simulink model "ThdRwLtStCaller"  (R2018b)
settings: Solver=FixedStepDiscrete  StartTime=0.0  StopTime=10.0  RelTol=1e-3
undefined symbols (not defined in the file): ThdRwLtStBkReclnCtrl_1_Cal, ThdRwLtStBkReclnHolderChk_1_Cal, ThdRwLtStBkReclnIsPosChk_1_Cal, ThdRwLtStBkReclnTrgtPosSelc_1_Cal, ThdRwLtStCshnFldCtrl_1_Cal, ThdRwLtStCshnFldHolderChk_1_Cal, ThdRwLtStCshnFldIsPosChk_1_Cal, ThdRwLtStCshnFldTrgtPosSelc_1_Cal, ThdRwLtStFwdBkwdCtrl_1_Cal, ThdRwLtStFwdBkwdHolderChk_1_Cal, ThdRwLtStFwdBkwdIsPosChk_1_Cal, ThdRwLtStFwdBkwdSpdCtrl_1_Cal, ThdRwLtStFwdBkwdTrgtPosSelc_1_Cal, ThdRwLtStRclCmdSrvCal_1_Cal
settings Model: Creator=sn2xws  LastModifiedBy=sn2xws
settings DataIOCC: SaveFormat=StructureWithTime
settings OptimizationCC: DefaultParameterBehavior=Inlined  EnhancedBackFolding=on  PassReuseOutputArgsAs=Individual arguments  ZeroExternalMemoryAtStartup=off  ZeroInternalMemoryAtStartup=off  OptimizeBlockOrder=speed  DifferentSizesBufferReuse=on  OptimizationCustomize=off
settings DebuggingCC: ParameterTunabilityLossMsg=error
settings SFSimCC: MATLABDynamicMemAlloc=off
settings RTWCC: SystemTargetFile=autosar.tlc  GenCodeOnly=on  TemplateMakefile=ert_default_tmf  Description=AUTOSAR  GenerateReport=on  IncludeHyperlinkInReport=on  LaunchReport=on  GenerateTraceInfo=on  GenerateTraceReport=on  GenerateTraceReportSl=on  GenerateTraceReportSf=on  GenerateTraceReportEml=on  GenerateCodeMetricsReport=on
settings CodeAppCC: ForceParamTrailComments=on  IgnoreCustomStorageClasses=off  OperatorAnnotations=on  SimulinkDataObjDesc=on  SFDataObjDesc=on  InsertBlockDesc=on
settings STFCustomTargetCC: TargetLangStandard=C99 (ISO)  MultiwordLength=256  ParMdlRefBuildCompliant=on  CompOptLevelCompliant=on  IncludeMdlTerminateFcn=off  CombineOutputUpdateFcns=on  SuppressErrorStatus=on  ERTCustomFileBanners=on  SupportNonFinite=off  SupportComplex=off  SupportContinuousTime=off  SupportNonInlinedSFcns=off  RemoveResetFunc=on  MATLABClassNameForMDSCustomization=Simulink.SoftwareTarget.ERTCustomization  AutosarCompliant=on  UseToolchainInfoCompliant=on  LookupTableObjectStructAxisOrder=2,1,3,4,...  LUTObjectStructOrderEvenSpacing=Size,Table,Breakpoints  SystemTargetFile=autosar.tlc
settings ERTTargetCC: TargetLangStandard=C99 (ISO)  ConcurrentExecutionCompliant=off  IncludeMdlTerminateFcn=off  SuppressErrorStatus=on  SupportNonFinite=off  SupportComplex=off  ModelStepFunctionPrototypeControlCompliant=off  CPPClassGenCompliant=off  AutosarCompliant=on  LookupTableObjectStructAxisOrder=2,1,3,4,...  LUTObjectStructOrderEvenSpacing=Size,Table,Breakpoints  InlinedParameterPlacement=NonHierarchical  ERTCustomFileTemplate=example_file_process.tlc  ERTFilePackagingFormat=Compact

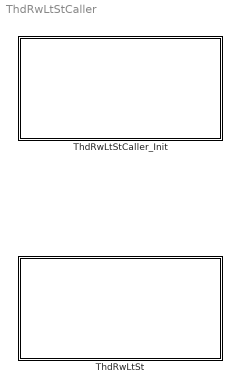
== system ThdRwLtStCaller ==
  ThdRwLtSt : Subsystem
  ThdRwLtStCaller_Init : Subsystem

== system ThdRwLtStCaller/ThdRwLtSt ==
  ThdRwLtSt_Cal_sys : Subsystem

== system ThdRwLtStCaller/ThdRwLtStCaller_Init ==
  Event Listener : EventListener  EventName=reset

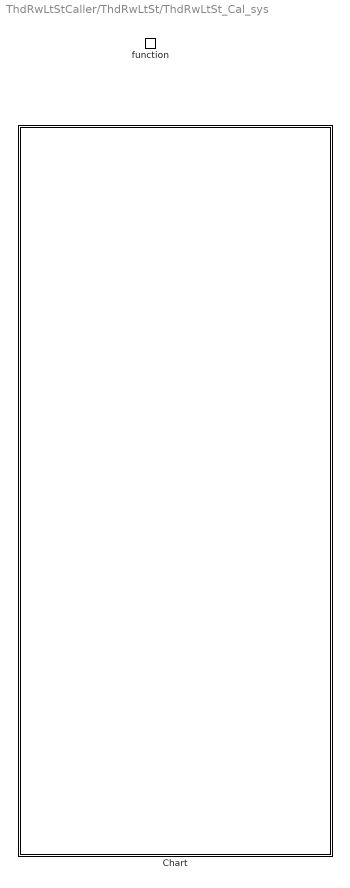
== system ThdRwLtStCaller/ThdRwLtSt/ThdRwLtSt_Cal_sys ==
  function : TriggerPort  TriggerType=function-call  IsSimulinkFunction=on  FunctionName=ThdRwLtSt_Cal  VariantControl=(inherit)
  Chart : Stateflow chart  TreatAsAtomicUnit=on

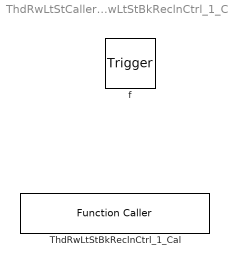
== system ThdRwLtStCaller/ThdRwLtSt/ThdRwLtSt_Cal_sys/Chart/ThdRwLtStBkReclnCtrl_1_Cal ==
  f : TriggerPort  TriggerType=function-call  VariantControl=(inherit)
      settings: CopyFcn=Stateflow.SLINSF.SimulinkMan.removeBlockPreDeleteFcn  PreDeleteFcn=Stateflow.SLINSF.SimulinkMan.unsafePredeleteFcn
  ThdRwLtStBkReclnCtrl_1_Cal : FunctionCaller  FunctionPrototype=ThdRwLtStBkReclnCtrl_1_Cal()

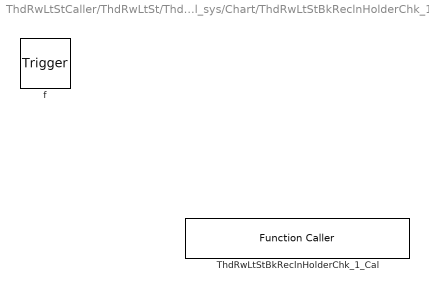
== system ThdRwLtStCaller/ThdRwLtSt/ThdRwLtSt_Cal_sys/Chart/ThdRwLtStBkReclnHolderChk_1_Cal ==
  f : TriggerPort  TriggerType=function-call  VariantControl=(inherit)
      settings: CopyFcn=Stateflow.SLINSF.SimulinkMan.removeBlockPreDeleteFcn  PreDeleteFcn=Stateflow.SLINSF.SimulinkMan.unsafePredeleteFcn
  ThdRwLtStBkReclnHolderChk_1_Cal : FunctionCaller  FunctionPrototype=ThdRwLtStBkReclnHolderChk_1_Cal()

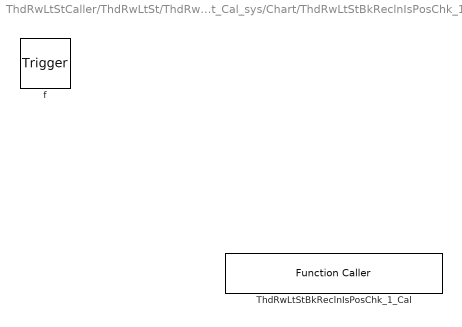
== system ThdRwLtStCaller/ThdRwLtSt/ThdRwLtSt_Cal_sys/Chart/ThdRwLtStBkReclnIsPosChk_1_Cal ==
  f : TriggerPort  TriggerType=function-call  VariantControl=(inherit)
      settings: CopyFcn=Stateflow.SLINSF.SimulinkMan.removeBlockPreDeleteFcn  PreDeleteFcn=Stateflow.SLINSF.SimulinkMan.unsafePredeleteFcn
  ThdRwLtStBkReclnIsPosChk_1_Cal : FunctionCaller  FunctionPrototype=ThdRwLtStBkReclnIsPosChk_1_Cal()

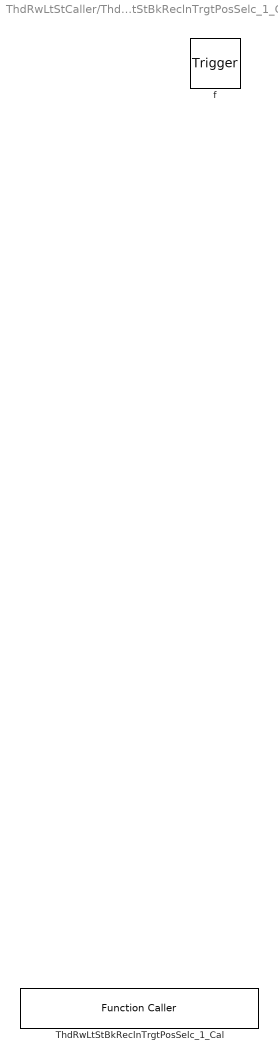
== system ThdRwLtStCaller/ThdRwLtSt/ThdRwLtSt_Cal_sys/Chart/ThdRwLtStBkReclnTrgtPosSelc_1_Cal ==
  f : TriggerPort  TriggerType=function-call  VariantControl=(inherit)
      settings: CopyFcn=Stateflow.SLINSF.SimulinkMan.removeBlockPreDeleteFcn  PreDeleteFcn=Stateflow.SLINSF.SimulinkMan.unsafePredeleteFcn
  ThdRwLtStBkReclnTrgtPosSelc_1_Cal : FunctionCaller  FunctionPrototype=ThdRwLtStBkReclnTrgtPosSelc_1_Cal()

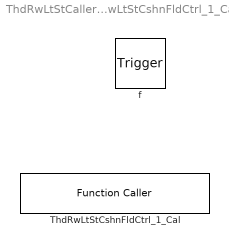
== system ThdRwLtStCaller/ThdRwLtSt/ThdRwLtSt_Cal_sys/Chart/ThdRwLtStCshnFldCtrl_1_Cal ==
  f : TriggerPort  TriggerType=function-call  VariantControl=(inherit)
      settings: CopyFcn=Stateflow.SLINSF.SimulinkMan.removeBlockPreDeleteFcn  PreDeleteFcn=Stateflow.SLINSF.SimulinkMan.unsafePredeleteFcn
  ThdRwLtStCshnFldCtrl_1_Cal : FunctionCaller  FunctionPrototype=ThdRwLtStCshnFldCtrl_1_Cal()

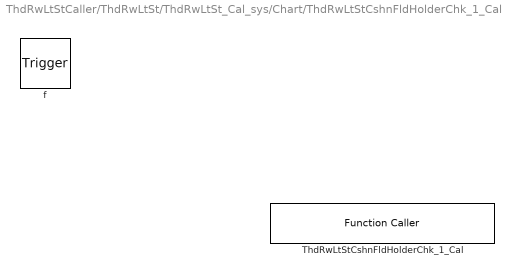
== system ThdRwLtStCaller/ThdRwLtSt/ThdRwLtSt_Cal_sys/Chart/ThdRwLtStCshnFldHolderChk_1_Cal ==
  f : TriggerPort  TriggerType=function-call  VariantControl=(inherit)
      settings: CopyFcn=Stateflow.SLINSF.SimulinkMan.removeBlockPreDeleteFcn  PreDeleteFcn=Stateflow.SLINSF.SimulinkMan.unsafePredeleteFcn
  ThdRwLtStCshnFldHolderChk_1_Cal : FunctionCaller  FunctionPrototype=ThdRwLtStCshnFldHolderChk_1_Cal()

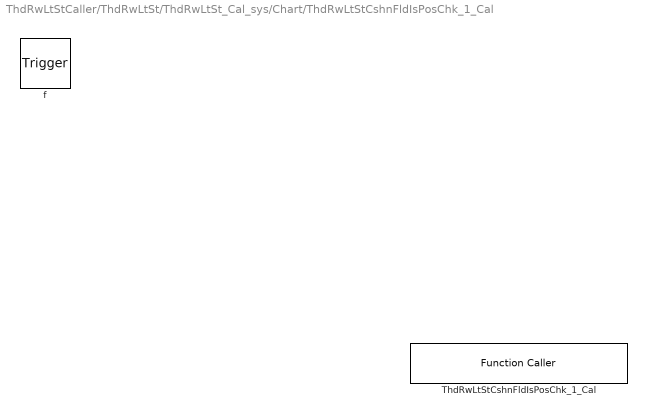
== system ThdRwLtStCaller/ThdRwLtSt/ThdRwLtSt_Cal_sys/Chart/ThdRwLtStCshnFldIsPosChk_1_Cal ==
  f : TriggerPort  TriggerType=function-call  VariantControl=(inherit)
      settings: CopyFcn=Stateflow.SLINSF.SimulinkMan.removeBlockPreDeleteFcn  PreDeleteFcn=Stateflow.SLINSF.SimulinkMan.unsafePredeleteFcn
  ThdRwLtStCshnFldIsPosChk_1_Cal : FunctionCaller  FunctionPrototype=ThdRwLtStCshnFldIsPosChk_1_Cal()

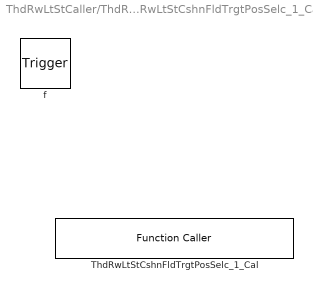
== system ThdRwLtStCaller/ThdRwLtSt/ThdRwLtSt_Cal_sys/Chart/ThdRwLtStCshnFldTrgtPosSelc_1_Cal ==
  f : TriggerPort  TriggerType=function-call  VariantControl=(inherit)
      settings: CopyFcn=Stateflow.SLINSF.SimulinkMan.removeBlockPreDeleteFcn  PreDeleteFcn=Stateflow.SLINSF.SimulinkMan.unsafePredeleteFcn
  ThdRwLtStCshnFldTrgtPosSelc_1_Cal : FunctionCaller  FunctionPrototype=ThdRwLtStCshnFldTrgtPosSelc_1_Cal()

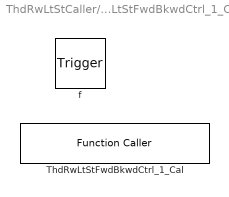
== system ThdRwLtStCaller/ThdRwLtSt/ThdRwLtSt_Cal_sys/Chart/ThdRwLtStFwdBkwdCtrl_1_Cal ==
  f : TriggerPort  TriggerType=function-call  VariantControl=(inherit)
      settings: CopyFcn=Stateflow.SLINSF.SimulinkMan.removeBlockPreDeleteFcn  PreDeleteFcn=Stateflow.SLINSF.SimulinkMan.unsafePredeleteFcn
  ThdRwLtStFwdBkwdCtrl_1_Cal : FunctionCaller  FunctionPrototype=ThdRwLtStFwdBkwdCtrl_1_Cal()

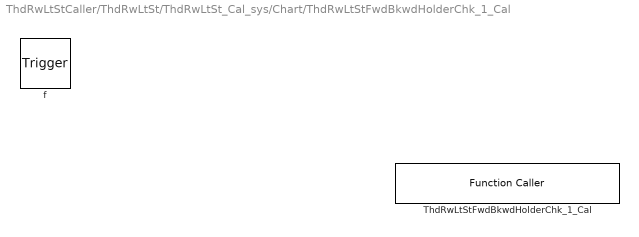
== system ThdRwLtStCaller/ThdRwLtSt/ThdRwLtSt_Cal_sys/Chart/ThdRwLtStFwdBkwdHolderChk_1_Cal ==
  f : TriggerPort  TriggerType=function-call  VariantControl=(inherit)
      settings: CopyFcn=Stateflow.SLINSF.SimulinkMan.removeBlockPreDeleteFcn  PreDeleteFcn=Stateflow.SLINSF.SimulinkMan.unsafePredeleteFcn
  ThdRwLtStFwdBkwdHolderChk_1_Cal : FunctionCaller  FunctionPrototype=ThdRwLtStFwdBkwdHolderChk_1_Cal()

== system ThdRwLtStCaller/ThdRwLtSt/ThdRwLtSt_Cal_sys/Chart/ThdRwLtStFwdBkwdIsPosChk_1_Cal ==
  f : TriggerPort  TriggerType=function-call  VariantControl=(inherit)
      settings: CopyFcn=Stateflow.SLINSF.SimulinkMan.removeBlockPreDeleteFcn  PreDeleteFcn=Stateflow.SLINSF.SimulinkMan.unsafePredeleteFcn
  ThdRwLtStFwdBkwdIsPosChk_1_Cal : FunctionCaller  FunctionPrototype=ThdRwLtStFwdBkwdIsPosChk_1_Cal()

== system ThdRwLtStCaller/ThdRwLtSt/ThdRwLtSt_Cal_sys/Chart/ThdRwLtStFwdBkwdSpdCtrl_1_Cal ==
  f : TriggerPort  TriggerType=function-call  VariantControl=(inherit)
      settings: CopyFcn=Stateflow.SLINSF.SimulinkMan.removeBlockPreDeleteFcn  PreDeleteFcn=Stateflow.SLINSF.SimulinkMan.unsafePredeleteFcn
  ThdRwLtStFwdBkwdSpdCtrl_1_Cal : FunctionCaller  FunctionPrototype=ThdRwLtStFwdBkwdSpdCtrl_1_Cal()

== system ThdRwLtStCaller/ThdRwLtSt/ThdRwLtSt_Cal_sys/Chart/ThdRwLtStFwdBkwdTrgtPosSelc_1_Cal ==
  f : TriggerPort  TriggerType=function-call  VariantControl=(inherit)
      settings: CopyFcn=Stateflow.SLINSF.SimulinkMan.removeBlockPreDeleteFcn  PreDeleteFcn=Stateflow.SLINSF.SimulinkMan.unsafePredeleteFcn
  ThdRwLtStFwdBkwdTrgtPosSelc_1_Cal : FunctionCaller  FunctionPrototype=ThdRwLtStFwdBkwdTrgtPosSelc_1_Cal()

== system ThdRwLtStCaller/ThdRwLtSt/ThdRwLtSt_Cal_sys/Chart/ThdRwLtStRclCmdSrvCal_1_Cal ==
  f : TriggerPort  TriggerType=function-call  VariantControl=(inherit)
      settings: CopyFcn=Stateflow.SLINSF.SimulinkMan.removeBlockPreDeleteFcn  PreDeleteFcn=Stateflow.SLINSF.SimulinkMan.unsafePredeleteFcn
  ThdRwLtStRclCmdSrvCal_1_Cal : FunctionCaller  FunctionPrototype=ThdRwLtStRclCmdSrvCal_1_Cal()

== stateflow chart ThdRwLtStCaller/ThdRwLtSt/ThdRwLtSt_Cal_sys/Chart ==
  state ThdRwLtStBkReclnTrgtPosSelc_1_Cal [function]
  state ThdRwLtStCshnFldTrgtPosSelc_1_Cal [function]
  state ThdRwLtStFwdBkwdTrgtPosSelc_1_Cal [function]
  state ThdRwLtStBkReclnIsPosChk_1_Cal [function]
  state ThdRwLtStCshnFldIsPosChk_1_Cal [function]
  state ThdRwLtStFwdBkwdIsPosChk_1_Cal [function]
  state ThdRwLtStBkReclnHolderChk_1_Cal [function]
  state ThdRwLtStCshnFldHolderChk_1_Cal [function]
  state ThdRwLtStFwdBkwdHolderChk_1_Cal [function]
  state ThdRwLtStBkReclnCtrl_1_Cal [function]
  state ThdRwLtStCshnFldCtrl_1_Cal [function]
  state ThdRwLtStFwdBkwdCtrl_1_Cal [function]
  state ThdRwLtStFwdBkwdSpdCtrl_1_Cal [function]
  state ThdRwLtStRclCmdSrvCal_1_Cal [function]
  (default) -> (junction 15)
  (junction 15) -> (junction 17) : {
      | ThdRwLtStBkReclnTrgtPosSelc_1_Cal();
      | ThdRwLtStCshnFldTrgtPosSelc_1_Cal();
      | ThdRwLtStFwdBkwdTrgtPosSelc_1_Cal();
      | ThdRwLtStBkReclnIsPosChk_1_Cal();
      | ThdRwLtStCshnFldIsPosChk_1_Cal();
      | ThdRwLtStFwdBkwdIsPosChk_1_Cal();
      | ThdRwLtStBkReclnHolderChk_1_Cal();
      | ThdRwLtStCshnFldHolderChk_1_Cal();
      | ThdRwLtStFwdBkwdHolderChk_1_Cal();
      | ThdRwLtStBkReclnCtrl_1_Cal();
      | ThdRwLtStCshnFldCtrl_1_Cal();
      | ThdRwLtStFwdBkwdCtrl_1_Cal();
      | ThdRwLtStFwdBkwdSpdCtrl_1_Cal();
      | ThdRwLtStRclCmdSrvCal_1_Cal();
      | }
